simulink model "DinamicaElaborato_final"  (R2023b)
settings: Solver=FixedStepAuto  StartTime=0.0  StopTime=60.0  FixedStep=0.005  RelTol=1e-3
undefined symbols (not defined in the file): Ki, Kp, Kv, magnitude, Q1r, Q2r
settings Model: Creator=franc  LastModifiedBy=franc
settings DebuggingCC: UnderSpecifiedDimensionMsg=warning

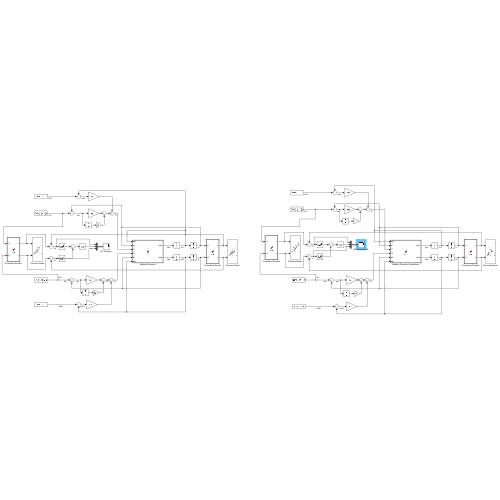
[thumbnail: Simulink's stored preview of the top-level diagram]
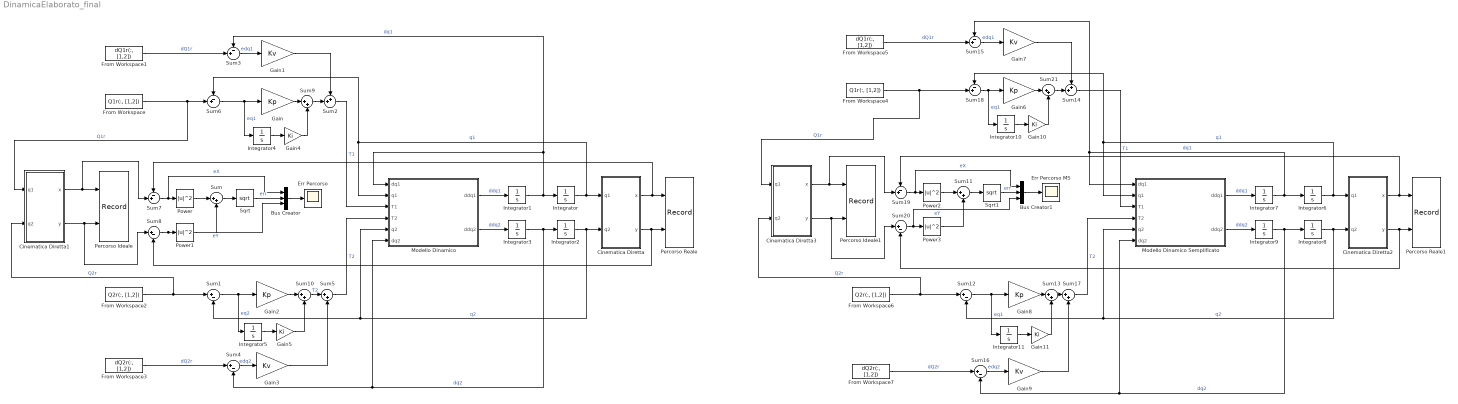
== system DinamicaElaborato_final ==
  Bus Creator : BusCreator  Inputs=3
  Bus Creator1 : BusCreator  Inputs=3
  Cinematica Diretta : MATLAB Function  TreatAsAtomicUnit=on
  Cinematica Diretta1 : MATLAB Function  TreatAsAtomicUnit=on
  Cinematica Diretta2 : MATLAB Function  TreatAsAtomicUnit=on
  Cinematica Diretta3 : MATLAB Function  TreatAsAtomicUnit=on
  Err Percorso : Scope
  Err Percorso MS : Scope
  From Workspace : FromWorkspace  VariableName=Q1r(:, [1,2])  OutputAfterFinalValue=Holding final value
  From Workspace1 : FromWorkspace  VariableName=dQ1r(:, [1,2])  OutputAfterFinalValue=Holding final value
  From Workspace2 : FromWorkspace  VariableName=Q2r(:, [1,2])  OutputAfterFinalValue=Holding final value
  From Workspace3 : FromWorkspace  VariableName=dQ2r(:, [1,2])  OutputAfterFinalValue=Holding final value
  From Workspace4 : FromWorkspace  VariableName=Q1r(:, [1,2])  OutputAfterFinalValue=Holding final value
  From Workspace5 : FromWorkspace  VariableName=dQ1r(:, [1,2])  OutputAfterFinalValue=Holding final value
  From Workspace6 : FromWorkspace  VariableName=Q2r(:, [1,2])  OutputAfterFinalValue=Holding final value
  From Workspace7 : FromWorkspace  VariableName=dQ2r(:, [1,2])  OutputAfterFinalValue=Holding final value
  Gain{,2,6,8} (4 alike) : Gain  Gain=Kp
  Gain{1,3,7,9} (4 alike) : Gain  Gain=Kv
  Gain{4..5,10..11} (4 alike) : Gain  Gain=Ki
  Integrator : Integrator  InitialCondition=Q1r(1,2)
  Integrator{1,3..5,7,9..11} (8 alike) : Integrator
  Integrator2 : Integrator  InitialCondition=Q2r(1,2)
  Integrator6 : Integrator  InitialCondition=Q1r(1,2)
  Integrator8 : Integrator  InitialCondition=Q2r(1,2)
  Modello Dinamico : MATLAB Function  TreatAsAtomicUnit=on
  Modello Dinamico Semplificato : MATLAB Function  TreatAsAtomicUnit=on
  Percorso Ideale : Record  FileSettingsInternal="{\"entries\":[{\"content\":{\"excelSettings\":{\"content\":{},\"type\":\"Streamout.ExcelSettings\"}},\"type\":\"Streamout.FileSettingStorage\",\"uuid\":\"\"}],\"packageUris\":[\"http:\\/\\/schema.mathworks.com\\/mf0\\/streamout_blocks\\/R2020a\"],\"version\":\"1.0\"}"  Layout=[1 1]  SignalsInternal="{\"entries\":[{\"content\":{\"signals\":[{\"content\":{\"blockPath\":[],\"dimensions\":[1],\"domain\":\"\",\"lineColor\":\"#64d413\",\"plots\":[1],\"port\":1,\"sid\":[\"\"],\"signalID\":162,\"signalName\":\"Cinematica Diretta1:1\"},\"type\":\"RecordBlkView.Signal\",\"uuid\":\"\"},{\"content\":{\"blockPath\":[],\"dimensions\":[1],\"domain\":\"\",\"lineColor\":\"#64d413\",\"plots\":[1],\"port\":2,\"sid\":[\"\"],\"signalID\":166,\"signalName\":\"Cinematica Diretta1:2\"},\"type\":\"RecordBlkView.Signal\",\"uuid\":\"\"}]},\"type\":\"RecordBlkView.InputSignals\",\"uuid\":\"\"}],\"packageUris\":[\"http:\\/\\/schema.mathworks.com\\/mf0\\/streamout_blocks\\/R2020a\"],\"version\":\"1.0\"}"  VisualizationBindings="{\"xyplotplugin\":{\"info\":[{\"series\":[{\"bindingParametersList\":[{\"parameter\":\"X-Axis\",\"signalID\":162,\"signalName\":\"Cinematica Diretta1:1\"},{\"parameter\":\"Y-Axis\",\"signalID\":166,\"signalName\":\"Cinematica Diretta1:2\"}],\"seriesID\":10805}],\"subplotID\":1}]}}"  CompatibilityTag=XY
  Percorso Ideale1 : Record  FileSettingsInternal="{\"entries\":[{\"content\":{\"excelSettings\":{\"content\":{},\"type\":\"Streamout.ExcelSettings\"}},\"type\":\"Streamout.FileSettingStorage\",\"uuid\":\"\"}],\"packageUris\":[\"http:\\/\\/schema.mathworks.com\\/mf0\\/streamout_blocks\\/R2020a\"],\"version\":\"1.0\"}"  Layout=[1 1]  SignalsInternal="{\"entries\":[{\"content\":{\"signals\":[{\"content\":{\"blockPath\":[],\"dimensions\":[1],\"domain\":\"\",\"lineColor\":\"#64d413\",\"plots\":[1],\"port\":1,\"sid\":[\"\"],\"signalID\":178,\"signalName\":\"Cinematica Diretta3:1\"},\"type\":\"RecordBlkView.Signal\",\"uuid\":\"\"},{\"content\":{\"blockPath\":[],\"dimensions\":[1],\"domain\":\"\",\"lineColor\":\"#64d413\",\"plots\":[1],\"port\":2,\"sid\":[\"\"],\"signalID\":182,\"signalName\":\"Cinematica Diretta3:2\"},\"type\":\"RecordBlkView.Signal\",\"uuid\":\"\"}]},\"type\":\"RecordBlkView.InputSignals\",\"uuid\":\"\"}],\"packageUris\":[\"http:\\/\\/schema.mathworks.com\\/mf0\\/streamout_blocks\\/R2020a\"],\"version\":\"1.0\"}"  VisualizationBindings="{\"xyplotplugin\":{\"info\":[{\"series\":[{\"bindingParametersList\":[{\"parameter\":\"X-Axis\",\"signalID\":178,\"signalName\":\"Cinematica Diretta3:1\"},{\"parameter\":\"Y-Axis\",\"signalID\":182,\"signalName\":\"Cinematica Diretta3:2\"}],\"seriesID\":53619}],\"subplotID\":1}]}}"  CompatibilityTag=XY
  Percorso Reale : Record  FileSettingsInternal="{\"entries\":[{\"content\":{\"excelSettings\":{\"content\":{},\"type\":\"Streamout.ExcelSettings\"}},\"type\":\"Streamout.FileSettingStorage\",\"uuid\":\"\"}],\"packageUris\":[\"http:\\/\\/schema.mathworks.com\\/mf0\\/streamout_blocks\\/R2020a\"],\"version\":\"1.0\"}"  Layout=[1 1]  SignalsInternal="{\"entries\":[{\"content\":{\"signals\":[{\"content\":{\"blockPath\":[],\"dimensions\":[1],\"domain\":\"\",\"lineColor\":\"#fe330a\",\"plots\":[1],\"port\":1,\"sid\":[\"\"],\"signalID\":170,\"signalName\":\"Cinematica Diretta:1\"},\"type\":\"RecordBlkView.Signal\",\"uuid\":\"\"},{\"content\":{\"blockPath\":[],\"dimensions\":[1],\"domain\":\"\",\"lineColor\":\"#fe330a\",\"plots\":[1],\"port\":2,\"sid\":[\"\"],\"signalID\":174,\"signalName\":\"Cinematica Diretta:2\"},\"type\":\"RecordBlkView.Signal\",\"uuid\":\"\"}]},\"type\":\"RecordBlkView.InputSignals\",\"uuid\":\"\"}],\"packageUris\":[\"http:\\/\\/schema.mathworks.com\\/mf0\\/streamout_blocks\\/R2020a\"],\"version\":\"1.0\"}"  VisualizationBindings="{\"xyplotplugin\":{\"info\":[{\"series\":[{\"bindingParametersList\":[{\"parameter\":\"X-Axis\",\"signalID\":170,\"signalName\":\"Cinematica Diretta:1\"},{\"parameter\":\"Y-Axis\",\"signalID\":174,\"signalName\":\"Cinematica Diretta:2\"}],\"seriesID\":29962}],\"subplotID\":1}]}}"  CompatibilityTag=XY
  Percorso Reale1 : Record  FileSettingsInternal="{\"entries\":[{\"content\":{\"excelSettings\":{\"content\":{},\"type\":\"Streamout.ExcelSettings\"}},\"type\":\"Streamout.FileSettingStorage\",\"uuid\":\"\"}],\"packageUris\":[\"http:\\/\\/schema.mathworks.com\\/mf0\\/streamout_blocks\\/R2020a\"],\"version\":\"1.0\"}"  Layout=[1 1]  SignalsInternal="{\"entries\":[{\"content\":{\"signals\":[{\"content\":{\"blockPath\":[],\"dimensions\":[1],\"domain\":\"\",\"lineColor\":\"#139fff\",\"plots\":[1],\"port\":1,\"sid\":[\"\"],\"signalID\":186,\"signalName\":\"Cinematica Diretta2:1\"},\"type\":\"RecordBlkView.Signal\",\"uuid\":\"\"},{\"content\":{\"blockPath\":[],\"dimensions\":[1],\"domain\":\"\",\"lineColor\":\"#139fff\",\"plots\":[1],\"port\":2,\"sid\":[\"\"],\"signalID\":190,\"signalName\":\"Cinematica Diretta2:2\"},\"type\":\"RecordBlkView.Signal\",\"uuid\":\"\"}]},\"type\":\"RecordBlkView.InputSignals\",\"uuid\":\"\"}],\"packageUris\":[\"http:\\/\\/schema.mathworks.com\\/mf0\\/streamout_blocks\\/R2020a\"],\"version\":\"1.0\"}"  VisualizationBindings="{\"xyplotplugin\":{\"info\":[{\"series\":[{\"bindingParametersList\":[{\"parameter\":\"X-Axis\",\"signalID\":186,\"signalName\":\"Cinematica Diretta2:1\"},{\"parameter\":\"Y-Axis\",\"signalID\":190,\"signalName\":\"Cinematica Diretta2:2\"}],\"seriesID\":17165}],\"subplotID\":1}]}}"  CompatibilityTag=XY
  Power{,1..3} (4 alike) : Math  Operator=magnitude^2  OutputSignalType=real
  Sqrt : Sqrt
  Sqrt1 : Sqrt
  Sum{,5,9..11,13,17,21} (8 alike) : Sum  Inputs=|++
  Sum{1,4,8,12,16,20} (6 alike) : Sum  Inputs=|+-
  Sum14 : Sum  Inputs=++|
  Sum{3,6..7,15,18..19} (6 alike) : Sum  Inputs=-+|
  Sum2 : Sum  Inputs=++|
  wires:
  Modello Dinamico/1(ddq1) -> Integrator1/1  "ddq1"
  Sum3/1 -> Gain1/1  "edq1"
  From Workspace/1 -> Cinematica Diretta1/1(q1), Sum6/2  "Q1r"
  Integrator1/1 -> Integrator/1, Modello Dinamico/1(dq1), Sum3/1  "dq1"
  Integrator/1 -> Sum6/1, Modello Dinamico/2(q1), Cinematica Diretta/1(q1)  "q1"
  Gain3/1 -> Sum5/2
  From Workspace2/1 -> Cinematica Diretta1/2(q2), Sum1/1  "Q2r"
  Sum4/1 -> Gain3/1  "edq2"
  From Workspace3/1 -> Sum4/1  "dQ2r"
  Cinematica Diretta/2(y) -> Sum8/2, Percorso Reale/2
  Cinematica Diretta/1(x) -> Percorso Reale/1, Sum7/1
  Integrator2/1 -> Sum1/2, Modello Dinamico/5(q2), Cinematica Diretta/2(q2)  "q2"
  Integrator3/1 -> Integrator2/1, Modello Dinamico/6(dq2), Sum4/2  "dq2"
  Modello Dinamico/2(ddq2) -> Integrator3/1  "ddq2"
  Sum5/1 -> Modello Dinamico/4(T2)  "T2"
  Sum2/1 -> Modello Dinamico/3(T1)  "T1"
  Cinematica Diretta1/1(x) -> Percorso Ideale/1, Sum7/2
  Cinematica Diretta1/2(y) -> Sum8/1, Percorso Ideale/2
  Sum7/1 -> Bus Creator/1, Power/1  "eX"
  Sum8/1 -> Bus Creator/3, Power1/1  "eY"
  Gain1/1 -> Sum2/1
  From Workspace1/1 -> Sum3/2  "dQ1r"
  Power/1 -> Sum/1
  Power1/1 -> Sum/2
  Sum/1 -> Sqrt/1
  Integrator4/1 -> Gain4/1
  Sum6/1 -> Integrator4/1, Gain/1  "eq1"
  Gain/1 -> Sum9/1
  Integrator5/1 -> Gain5/1
  Sum1/1 -> Integrator5/1, Gain2/1  "eq2"
  Sum9/1 -> Sum2/2
  Gain4/1 -> Sum9/2
  Gain2/1 -> Sum10/1
  Sum10/1 -> Sum5/1  "T2"
  Gain5/1 -> Sum10/2
  Bus Creator/1 -> Err Percorso/1
  Sqrt/1 -> Bus Creator/2  "err"
  Sum12/1 -> Gain8/1, Integrator11/1  "eq1"
  Cinematica Diretta2/2(y) -> Percorso Reale1/2, Sum20/2
  From Workspace4/1 -> Sum18/2, Cinematica Diretta3/1(q1)  "Q1r"
  Sqrt1/1 -> Bus Creator1/2  "err"
  Sum13/1 -> Sum17/1
  Gain8/1 -> Sum13/1
  Cinematica Diretta2/1(x) -> Percorso Reale1/1, Sum19/1
  Integrator9/1 -> Integrator8/1, Modello Dinamico Semplificato/6(dq2), Sum16/2  "dq2"
  From Workspace7/1 -> Sum16/1  "dQ2r"
  Sum21/1 -> Sum14/2
  Integrator10/1 -> Gain10/1
  From Workspace5/1 -> Sum15/2  "dQ1r"
  Power3/1 -> Sum11/2
  Power2/1 -> Sum11/1
  Gain11/1 -> Sum13/2
  Gain6/1 -> Sum21/1
  Sum19/1 -> Bus Creator1/1, Power2/1  "eX"
  Gain9/1 -> Sum17/2
  Integrator6/1 -> Sum18/1, Modello Dinamico Semplificato/2(q1), Cinematica Diretta2/1(q1)  "q1"
  Integrator11/1 -> Gain11/1
  Gain7/1 -> Sum14/1
  Bus Creator1/1 -> Err Percorso MS/1
  Cinematica Diretta3/2(y) -> Sum20/1, Percorso Ideale1/2
  Cinematica Diretta3/1(x) -> Percorso Ideale1/1, Sum19/2
  Sum20/1 -> Bus Creator1/3, Power3/1  "eY"
  Integrator7/1 -> Integrator6/1, Modello Dinamico Semplificato/1(dq1), Sum15/1  "dq1"
  Sum14/1 -> Modello Dinamico Semplificato/3(T1)  "T1"
  Sum15/1 -> Gain7/1  "edq1"
  From Workspace6/1 -> Cinematica Diretta3/2(q2), Sum12/1  "Q2r"
  Sum18/1 -> Integrator10/1, Gain6/1  "eq1"
  Gain10/1 -> Sum21/2
  Sum16/1 -> Gain9/1  "edq2"
  Sum11/1 -> Sqrt1/1
  Sum17/1 -> Modello Dinamico Semplificato/4(T2)  "T2"
  Modello Dinamico Semplificato/1(ddq1) -> Integrator7/1  "ddq1"
  Integrator8/1 -> Modello Dinamico Semplificato/5(q2), Sum12/2, Cinematica Diretta2/2(q2)  "q2"
  Modello Dinamico Semplificato/2(ddq2) -> Integrator9/1  "ddq2"

== matlab function DinamicaElaborato_final/Cinematica Diretta ==
  data: q1 input; x output; q2 input; y output
function [x, y]= fcn(q1,q2)
L1=1;
L2=1;

c1=cos(q1);
c12=cos(q1+q2);
s1=sin(q1);
s12=sin(q1+q2);

x=L1*c1+L2*c12;
y=L1*s1+L2*s12;

== matlab function DinamicaElaborato_final/Modello Dinamico ==
  data: dq1 input; q1 input; T1 input; T2 input; q2 input; ddq1 output; dq2 input; ddq2 output
function [ddq1,ddq2]= fcn(dq1,q1,T1,T2,q2,dq2)
g=9.81;
Q=[q1;q2];
dQ=[dq1;dq2];
T=[T1;T2];

a1=1;
a2=1;
m1=1;
m2=1;
l1=a1/2;
l2=a2/2;
I1=m1*a1^2/12;
I2=m2*a2^2/12;

c1=cos(q1);
c2=cos(q2);
s2=sin(q2);

% Matrice di Inerzia
    M=[(m1*l1^2 +I1+m2*a1^2+m2*l2^2 +2*m2*a1*l2*c2+I2), (m2*l2^2 + m2*a1*l2*c2+I2);
          (m2*l1^2 +m2*a1*l2*c2+I2), (m2*l2^2 +I2)];

% Matrice delle Forze Apparenti
    H=[-2*m2*a1*l2*s2*dq2, -m2*a1*l2*s2*dq2;
          m2*a1*l2*s2*dq1, 0];
    
    % Termini Gravitazionali
    G=[(m1*l1+m2*a1)*g*c1+m2*g*l2*cos(q1+q2); m2*g*l2*cos(q1+q2)];


ddQ = inv(M)*T - inv(M)*H*dQ - inv(M)*G;


ddq1=ddQ(1);
ddq2=ddQ(2);

== matlab function DinamicaElaborato_final/Cinematica Diretta1 ==
  data: q1 input; x output; q2 input; y output
function [x, y]= fcn(q1,q2)
L1=1;
L2=1;

c1=cos(q1);
c12=cos(q1+q2);
s1=sin(q1);
s12=sin(q1+q2);

x=L1*c1+L2*c12;
y=L1*s1+L2*s12;

== matlab function DinamicaElaborato_final/Cinematica Diretta2 ==
  data: q1 input; x output; q2 input; y output
function [x, y]= fcn(q1,q2)
L1=1;
L2=1;

c1=cos(q1);
c12=cos(q1+q2);
s1=sin(q1);
s12=sin(q1+q2);

x=L1*c1+L2*c12;
y=L1*s1+L2*s12;

== matlab function DinamicaElaborato_final/Cinematica Diretta3 ==
  data: q1 input; x output; q2 input; y output
function [x, y]= fcn(q1,q2)
L1=1;
L2=1;

c1=cos(q1);
c12=cos(q1+q2);
s1=sin(q1);
s12=sin(q1+q2);

x=L1*c1+L2*c12;
y=L1*s1+L2*s12;

== matlab function DinamicaElaborato_final/Modello Dinamico Semplificato ==
  data: dq1 input; q1 input; T1 input; T2 input; q2 input; ddq1 output; dq2 input; ddq2 output
function [ddq1,ddq2]= fcn(dq1,q1,T1,T2,q2,dq2)
g=1.2;
Q=[q1;q2];
dQ=[dq1;dq2];
T=[T1;T2];

a1=1;
a2=1;
m1=1;
m2=1;
l1=a1/2;
l2=a2/2;
I1=m1*a1^2/12;
I2=m2*a2^2/12;

c1=cos(q1);
c2=cos(q2);
s2=sin(q2);

% Matrice di Inerzia
    M=[(m1*l1^2 +I1+m2*a1^2+m2*l2^2 +2*m2*a1*l2*c2+I2), (m2*l2^2 + m2*a1*l2*c2+I2);
          (m2*l1^2 +m2*a1*l2*c2+I2), (m2*l2^2 +I2)];
    
    % Termini Gravitazionali
    G=[(m1*l1+m2*a1)*g*c1+m2*g*l2*cos(q1+q2); m2*g*l2*cos(q1+q2)];


ddQ = inv(M)*T - inv(M)*G;


ddq1=ddQ(1);
ddq2=ddQ(2);
